simulink model "productionLine"  (R2023a)
settings: Solver=VariableStepAuto  StartTime=0.0  StopTime=10.0  RelTol=1e-3
libraries: NSA_DEVS_SINKS x8, ProductionLineLib_CM x7, NSA_DEVS_LOGISTICS x2, NSA_DEVS_SOURCES x1
settings Model: Creator=peter  LastModifiedBy=peter

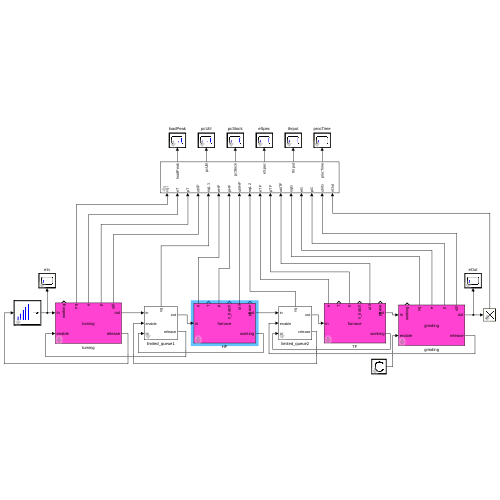
[thumbnail: Simulink's stored preview of the top-level diagram]
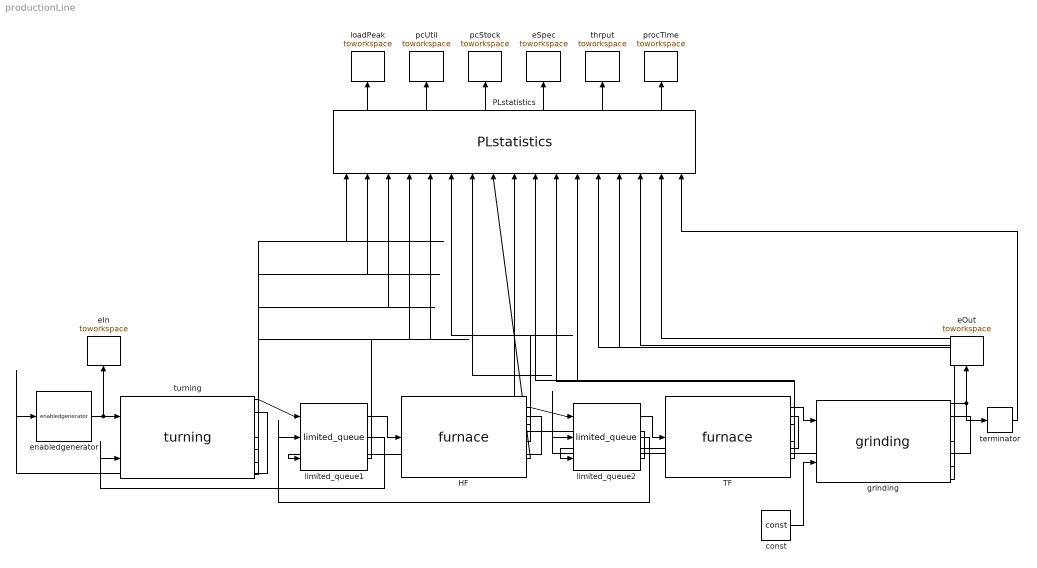
== system productionLine ==
  HF : ProductionLineLib_CM/furnace  PH=20000  Co=12000  k_A=10  Te=25  P0=2000  P_unload=120000  holding_time=1800*3  Tsoll=800  Kapa=70  tauInt=[0,1]  tauCont=[0,1]  tau=[0,1]  debug=0
      link override unbatch: tau=[0,1]  tD=[0,2]
  PLstatistics : ProductionLineLib_CM/PLstatistics  tau=[0,1]  debug=0
  TF : ProductionLineLib_CM/furnace  PH=20000  Co=12000  k_A=10  Te=25  P0=2000  P_unload=50000  holding_time=3600*3  Tsoll=400  Kapa=70  tauInt=[0,1]  tauCont=[0,1]  tau=[0,1]  debug=0
      link override unbatch: tau=[0,1]  tD=[0,6]
  const : NSA_DEVS_SOURCES/const  value=1  sendTime=[0,1]  tau=[0,1]  debug=0
      settings: SourceProductName=NSA_DEVS
  eIn : NSA_DEVS_SINKS/toworkspace  varname="\"eIn\""  t0=0  format="\"vector\""  tau=[0,1]  debug=0
      settings: SourceProductName=NSA_DEVS
  eOut : NSA_DEVS_SINKS/toworkspace  varname="\"eOut\""  t0=0  format="\"vector\""  tau=[0,1]  debug=0
      settings: SourceProductName=NSA_DEVS
  eSpec : NSA_DEVS_SINKS/toworkspace  varname="\"eSpec\""  t0=0  format="\"vector\""  tau=[0,1]  debug=0
      settings: SourceProductName=NSA_DEVS
  enabledgenerator : NSA_DEVS_LOGISTICS/enabledgenerator  tG=5*60  n0=1  nG=560  tau=[0,1]  debug=0
      settings: SourceProductName=NSA_DEVS
  grinding : ProductionLineLib_CM/grinding  vfr1=0.48  vfr2=0.19  vfr3=0.03  vc=30  max_fifo=400  tauInt=[0,1]  tauCont=[0,1]  tau=[0,1]  debug=0
      link override combine3: tD=[0,2]
      link override input_queue: tau=[0,1]  tD=[0,2]
      link override input_queue/distribute3: tau=[0,1]
  limited_queue1 : ProductionLineLib_CM/limited_queue  max_fifo=400  tD=[0,2]  tau=[0,1]  debug=0
  limited_queue2 : ProductionLineLib_CM/limited_queue  max_fifo=400  tD=[0,2]  tau=[0,1]  debug=0
  loadPeak : NSA_DEVS_SINKS/toworkspace  varname="\"loadPeak\""  t0=0  format="\"vector\""  tau=[0,1]  debug=0
      settings: SourceProductName=NSA_DEVS
  pcStock : NSA_DEVS_SINKS/toworkspace  varname="\"pcStock\""  t0=0  format="\"vector\""  tau=[0,1]  debug=0
      settings: SourceProductName=NSA_DEVS
  pcUtil : NSA_DEVS_SINKS/toworkspace  varname="\"pcUtil\""  t0=0  format="\"vector\""  tau=[0,1]  debug=0
      settings: SourceProductName=NSA_DEVS
  procTime : NSA_DEVS_SINKS/toworkspace  varname="\"procTime\""  t0=0  format="\"vector\""  tau=[0,1]  debug=0
      settings: SourceProductName=NSA_DEVS
  terminator : NSA_DEVS_LOGISTICS/terminator  tau=[0,1]  debug=0
      settings: SourceProductName=NSA_DEVS
  thrput : NSA_DEVS_SINKS/toworkspace  varname="\"thrput\""  t0=0  format="\"vector\""  tau=[0,1]  debug=0
      settings: SourceProductName=NSA_DEVS
  turning : ProductionLineLib_CM/turning  ap=0.5  f=0.1  vc=150  max_fifo=400  tauInt=[0,1]  tauCont=[0,1]  tau=[0,1]  debug=0
      link override combine3: tD=[0,2]
      link override input_queue: tau=[0,1]  tD=[0,2]
      link override input_queue/distribute3: tau=[0,1]
  wires:
  enabledgenerator/1 -> eIn/1, turning/1
  turning/1 -> limited_queue1/1
  limited_queue1/1 -> HF/1
  HF/1 -> limited_queue2/1
  limited_queue2/1 -> TF/1
  TF/1 -> grinding/1
  grinding/1 -> eOut/1, terminator/1
  limited_queue1/2 -> turning/2
  limited_queue2/2 -> limited_queue1/2
  HF/2 -> limited_queue1/3
  grinding/2 -> limited_queue2/2
  TF/2 -> limited_queue2/3
  const/1 -> grinding/2
  turning/4 -> PLstatistics/1
  turning/5 -> PLstatistics/2
  turning/6 -> PLstatistics/3
  turning/7 -> PLstatistics/4
  terminator/1 -> PLstatistics/17
  PLstatistics/1 -> loadPeak/1
  PLstatistics/2 -> pcUtil/1
  PLstatistics/3 -> pcStock/1
  PLstatistics/4 -> eSpec/1
  limited_queue1/3 -> PLstatistics/5
  HF/3 -> PLstatistics/6
  HF/5 -> PLstatistics/7
  HF/7 -> PLstatistics/8
  limited_queue2/3 -> PLstatistics/9
  TF/3 -> PLstatistics/10
  TF/5 -> PLstatistics/11
  TF/7 -> PLstatistics/12
  grinding/4 -> PLstatistics/13
  grinding/5 -> PLstatistics/14
  grinding/6 -> PLstatistics/15
  grinding/7 -> PLstatistics/16
  PLstatistics/5 -> thrput/1
  PLstatistics/6 -> procTime/1
  turning/2 -> enabledgenerator/1
